simulink model "SVPWM_model"  (R2023a)
settings: Solver=ode1  StartTime=0.0  StopTime=0.4  FixedStep=0.000001  RelTol=1e-3
InitFcn:
  | Vdc=1;
libraries: simulink_extras x1, simulink x1
settings Model: Creator=Lei  LastModifiedBy=Guoguo
settings SolverCC: AlgebraicLoopSolver=TrustRegion
settings DataIOCC: SaveFormat=Array  SignalLoggingSaveFormat=ModelDataLogs  SaveOutput=off  ReturnWorkspaceOutputs=off  TimeSaveName=t  SignalLoggingName=sigsOut
settings OptimizationCC: BlockReduction=off  BooleanDataType=off  ExpressionDepthLimit=2147483647  LifeSpan=inf
settings DebuggingCC: SaveWithParameterizedLinksMsg=none  UnderspecifiedInitializationDetection=Classic  MergeDetectMultiDrivingBlocksExec=none  SignalResolutionControl=TryResolveAllWithWarning  MultiTaskDSMMsg=warning  MultiTaskCondExecSysMsg=none  FcnCallInpInsideContextMsg=warning  UnconnectedInputMsg=warning  UnconnectedOutputMsg=warning  UnconnectedLineMsg=warning  StateNameClashWarn=warning  SFUnexpectedBacktrackingDiag=warning  SFNoUnconditionalDefaultTransitionDiag=warning  SFExecutionAtInitializationDiag=none  ArithmeticOperatorsInVariantConditions=warning
settings HardwareCC: ProdBitPerPointer=32  ProdBitPerSizeT=32  ProdBitPerPtrDiffT=32  ProdLargestAtomicFloat=None  ProdIntDivRoundTo=Undefined  ProdEndianess=Unspecified  ProdWordSize=32  ProdHWDeviceType=32-bit Generic  TargetUnknown=on
settings ModelReferenceCC: PropagateSignalLabelsOutOfModel=off
settings SFSimCC: SimUseLocalCustomCode=off  SimParseCustomCode=off  CustomCodeUndefinedFunction=UseInterfaceOnly
settings RTWCC: RTWUseLocalCustomCode=off
settings CodeAppCC: StateflowObjectComments=on
settings GRTTargetCC: TargetLangStandard=C89/C90 (ANSI)  CombineOutputUpdateFcns=off  GRTInterface=on
settings ConfigComp: CovMetricSettings=dw  CovSaveCumulativeToWorkspaceVar=on  CovSaveSingleToWorkspaceVar=on  CovExternalEMLEnable=off

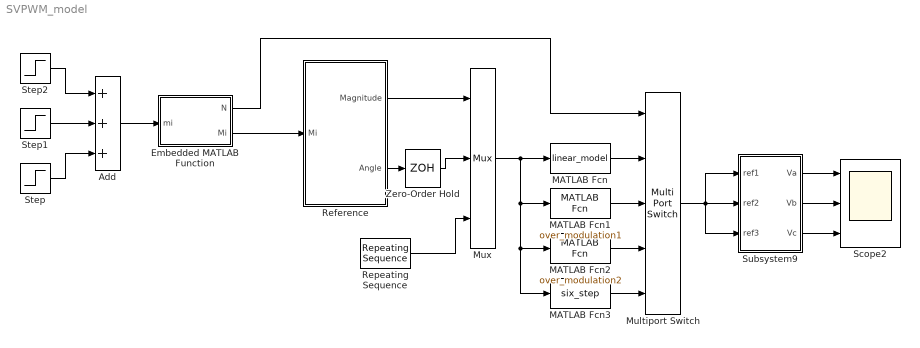
== system SVPWM_model ==
  Add : Sum  Inputs=+++
  Embedded MATLAB Function : MATLAB Function  TreatAsAtomicUnit=on
  MATLAB Fcn : MATLABFcn  MATLABFcn=linear_model  OutputDimensions=3
  MATLAB Fcn1 : MATLABFcn  MATLABFcn=over_modulation1  OutputDimensions=3
  MATLAB Fcn2 : MATLABFcn  MATLABFcn=over_modulation2  OutputDimensions=3
  MATLAB Fcn3 : MATLABFcn  MATLABFcn=six_step  OutputDimensions=3
  Multiport Switch : MultiPortSwitch  Inputs=4  SaturateOnIntegerOverflow=off  InputSameDT=off
  Mux : Mux  Inputs=3
  Reference : Subsystem
  Repeating Sequence : simulink/Sources/Repeating Sequence  rep_seq_t=[0 0.0002]  rep_seq_y=[0 0.0002]
  Scope2 : Scope  NumInputPorts=3
  Step : Step  Time=0.1  Before=0.455  After=0.544  SampleTime=0
  Step1 : Step  Time=0.2  Before=0.036  After=0.076  SampleTime=0
  Step2 : Step  Time=0.3  Before=0.012  After=2/pi-0.62  SampleTime=0
  Subsystem9 : Subsystem
      mask Display:
      | disp('3-Ph\nVSI')
      | port_label('input',1,'Sa')
      | port_label('input',2,'Sb')
      | port_label('input',3,'Se')
      | port_label('output',1,'Va')
      | port_label('output',2,'Vb')
      | port_label('output',3,'Ve')
  Zero-Order Hold : ZeroOrderHold  SampleTime=0.0002
  wires:
  Reference/1(Magnitude) -> Mux/1
  Reference/2(Angle) -> Zero-Order Hold/1
  Zero-Order Hold/1 -> Mux/2
  Mux/1 -> MATLAB Fcn/1, MATLAB Fcn1/1, MATLAB Fcn2/1, MATLAB Fcn3/1
  Repeating Sequence/1 -> Mux/3
  Subsystem9/1(Va) -> Scope2/1
  Subsystem9/2(Vb) -> Scope2/2
  Subsystem9/3(Vc) -> Scope2/3
  Step/1 -> Add/3
  Step1/1 -> Add/2
  Add/1 -> Embedded MATLAB Function/1(mi)
  Step2/1 -> Add/1
  MATLAB Fcn/1 -> Multiport Switch/2
  MATLAB Fcn1/1 -> Multiport Switch/3
  MATLAB Fcn2/1 -> Multiport Switch/4
  MATLAB Fcn3/1 -> Multiport Switch/5
  Embedded MATLAB Function/1(N) -> Multiport Switch/1
  Multiport Switch/1 -> Subsystem9/1(ref1), Subsystem9/2(ref2), Subsystem9/3(ref3)
  Embedded MATLAB Function/2(Mi) -> Reference/1(Mi)

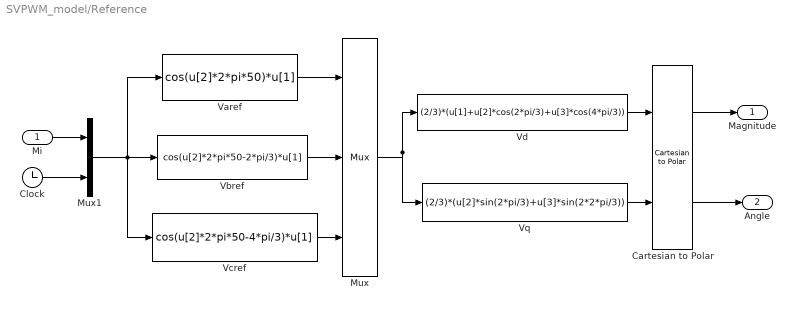
== system SVPWM_model/Reference ==
  Mi : Inport
  Cartesian to Polar : simulink_extras/Transformations/Cartesian to Polar
  Clock : Clock
  Mux : Mux  Inputs=3
  Mux1 : Mux  Inputs=2
  Varef : Fcn  Expr=cos(u[2]*2*pi*50)*u[1]
  Vbref : Fcn  Expr=cos(u[2]*2*pi*50-2*pi/3)*u[1]
  Vcref : Fcn  Expr=cos(u[2]*2*pi*50-4*pi/3)*u[1]
  Vd : Fcn  Expr=(2/3)*(u[1]+u[2]*cos(2*pi/3)+u[3]*cos(4*pi/3))
  Vq : Fcn  Expr=(2/3)*(u[2]*sin(2*pi/3)+u[3]*sin(2*2*pi/3))
  Magnitude : Outport
  Angle : Outport  Port=2
  wires:
  Varef/1 -> Mux/1
  Vbref/1 -> Mux/2
  Vcref/1 -> Mux/3
  Mux/1 -> Vd/1, Vq/1
  Vd/1 -> Cartesian to Polar/1
  Vq/1 -> Cartesian to Polar/2
  Cartesian to Polar/1 -> Magnitude/1
  Cartesian to Polar/2 -> Angle/1
  Mux1/1 -> Vbref/1, Varef/1, Vcref/1
  Clock/1 -> Mux1/2
  Mi/1 -> Mux1/1

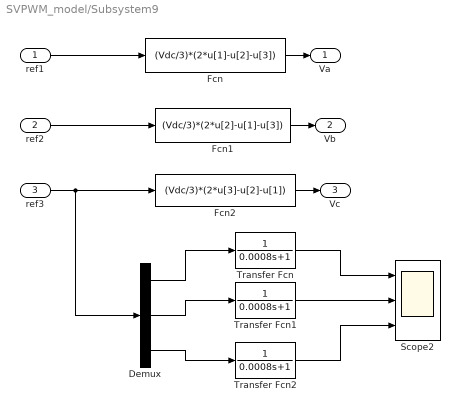
== system SVPWM_model/Subsystem9 ==
  ref1 : Inport
  ref2 : Inport  Port=2
  ref3 : Inport  Port=3
  Demux : Demux  Outputs=3
      settings: DisplayOption=none
  Fcn : Fcn  Expr=(Vdc/3)*(2*u[1]-u[2]-u[3])
  Fcn1 : Fcn  Expr=(Vdc/3)*(2*u[2]-u[1]-u[3])
  Fcn2 : Fcn  Expr=(Vdc/3)*(2*u[3]-u[2]-u[1])
  Scope2 : Scope  NumInputPorts=3
  Transfer Fcn : TransferFcn  Denominator=[0.0008 1]
  Transfer Fcn1 : TransferFcn  Denominator=[0.0008 1]
  Transfer Fcn2 : TransferFcn  Denominator=[0.0008 1]
  Va : Outport
  Vb : Outport  Port=2
  Vc : Outport  Port=3
  wires:
  Fcn/1 -> Va/1
  Fcn1/1 -> Vb/1
  Fcn2/1 -> Vc/1
  ref1/1 -> Fcn/1
  ref2/1 -> Fcn1/1
  ref3/1 -> Fcn2/1, Demux/1
  Demux/1 -> Transfer Fcn/1
  Demux/2 -> Transfer Fcn1/1
  Demux/3 -> Transfer Fcn2/1
  Transfer Fcn/1 -> Scope2/1
  Transfer Fcn1/1 -> Scope2/2
  Transfer Fcn2/1 -> Scope2/3

== matlab function SVPWM_model/Embedded MATLAB Function ==
  data: mi input; N output; Mi output
function [N,Mi] = fcn(mi)
%#eml
if mi<=0.5773
    N =1;
    Mi = mi;
elseif mi<=0.6061
    N =2;
    Mi = mi;
elseif mi<0.6366
    N =3;
    Mi = mi;
else
     N =4;
     Mi = mi;
end
end
